simulink model "FEDNNSimulacion"  (R2022b)
settings: Solver=ode1be  StartTime=0.0  StopTime=30  FixedStep=0.01  RelTol=1e-3
undefined symbols (not defined in the file): A, B, f, ne
settings Model: Creator=raul  LastModifiedBy=raul

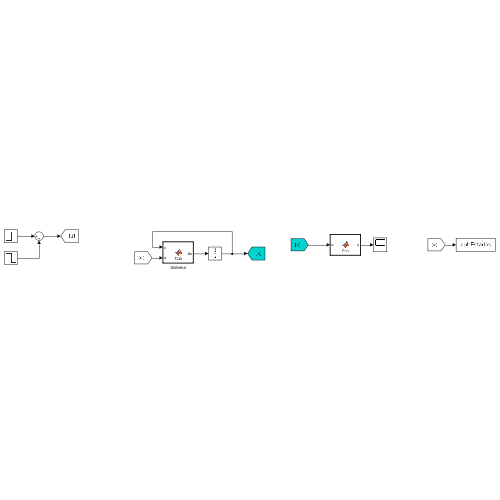
[thumbnail: Simulink's stored preview of the top-level diagram]
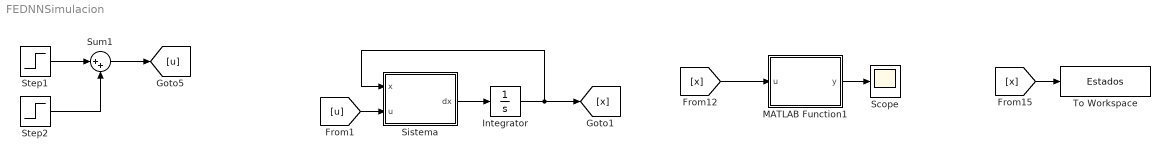
== system FEDNNSimulacion ==
  Integrator : Integrator  InitialCondition=zeros(2*ne,ne)
  MATLAB Function1 : MATLAB Function  TreatAsAtomicUnit=on
  Scope : Scope
  Sistema : MATLAB Function  TreatAsAtomicUnit=on
  Step1 : Step  SampleTime=0
  Step2 : Step  Time=1.1  After=-1  SampleTime=0
  Sum1 : Sum  Inputs=|++
  To Workspace : ToWorkspace  VariableName=Estados  SampleTime=-1
  wires:
  Step2/1 -> Sum1/2
  Step1/1 -> Sum1/1
  Sistema/1(dx) -> Integrator/1
  Integrator/1 -> [x], Sistema/1(x)
  Sum1/1 -> [u]
  [u] -> Sistema/2(u)
  MATLAB Function1/1(y) -> Scope/1
  [x] -> MATLAB Function1/1(u)
  [x] -> To Workspace/1

== matlab function FEDNNSimulacion/Sistema ==
  data: x input; u input; dx output; A parameter; B parameter; f parameter
function dx = fcn(x,u,A, B, f)%add Bw,w

dx = A*x+B*u;

%dx = A*x+B(:,f)*u+Bw*w;

== matlab function FEDNNSimulacion/MATLAB Function1 ==
  data: u input; y output; f parameter
function y = fcn(u,f)

y = u(:,f);
